simulink model "compiled_model"  (R2021a)
settings: Solver=VariableStepAuto  StartTime=0.0  StopTime=120  RelTol=1e-3
undefined symbols (not defined in the file or in its folder): sigbuilder_block
libraries: fuzblock x1, mpcadaslib x1
settings Model: Creator=uddin  LastModifiedBy=uddin

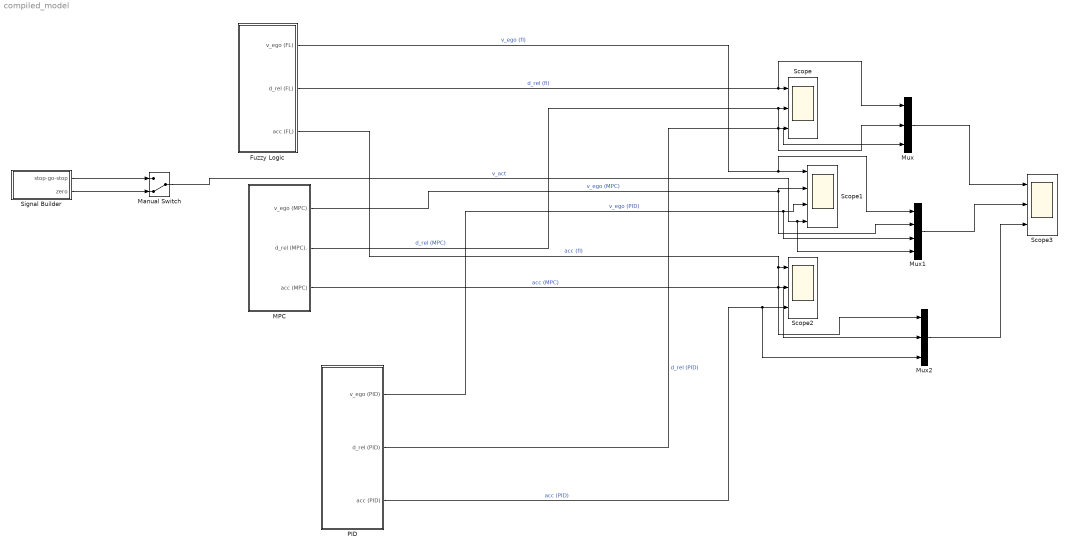
== system compiled_model ==
  Fuzzy Logic : Subsystem
  MPC : Subsystem
  Manual Switch : ManualSwitch  CurrentSetting=0
  Mux : Mux  Inputs=3
  Mux1 : Mux
  Mux2 : Mux  Inputs=3
  PID : Subsystem
  Scope : Scope  NumInputPorts=3
  Scope1 : Scope  NumInputPorts=4
  Scope2 : Scope  NumInputPorts=3
  Scope3 : Scope  NumInputPorts=3
  Signal Builder : Subsystem  Tag=STV Subsys  LoadFcn=sigbuilder_block('load');  StartFcn=sigbuilder_block('start');  StopFcn=sigbuilder_block('stop');  ClipboardFcn=sigbuilder_block('clipboard');  mask(Sigbuilder block){tuvar=[0:10]}
      mask help: Simulink:masks:SigbuilderBlock_MD
      mask init:
      | if ~strcmp(get_param(bdroot(gcbh),'SimulationStatus'),'stopped') tuvar = sigbuilder_block('maskInit'); end
      settings: CopyFcn=sigbuilder_block('copy');  DeleteFcn=sigbuilder_block('delete');  ModelCloseFcn=sigbuilder_block('modelClose');  PreSaveFcn=sigbuilder_block('preSave');  PauseFcn=sigbuilder_block('pause');  ContinueFcn=sigbuilder_block('continue');  NameChangeFcn=sigbuilder_block('namechange');  OpenFcn=sigbuilder_block('open',[393 134.4 550.8 400.2 ]);  CloseFcn=sigbuilder_block('close');
      mask Display: plot(0, 0, 100, 100,[2, 2, 32, 32, 2], [68, 8, 8, 68, 68],[32, 2], [38, 38], [32, 19, 2],[53, 60, 44], [32, 17, 17, 2],[16, 16, 31, 31]);txt = getActiveGroup(gcbh);text(2, 100, txt,'verticalAlignment', 'top');
  wires:
  Fuzzy Logic/2(d_rel (FL)) -> Mux/1, Scope/1  "d_rel (fl)"
  MPC/2(d_rel (MPC).) -> Mux/2, Scope/2  "d_rel (MPC)"
  PID/2(d_rel (PID)) -> Mux/3, Scope/3  "d_rel (PID)"
  Fuzzy Logic/1(v_ego (FL)) -> Mux1/1, Scope1/1  "v_ego (fl)"
  MPC/1(v_ego (MPC)) -> Mux1/2, Scope1/2  "v_ego (MPC)"
  PID/1(v_ego (PID)) -> Mux1/3, Scope1/3  "v_ego (PID)"
  Fuzzy Logic/3(acc (FL)) -> Mux2/1, Scope2/1  "acc (fl)"
  MPC/3(acc (MPC)) -> Mux2/2, Scope2/2  "acc (MPC)"
  PID/3(acc (PID)) -> Scope2/3, Mux2/3  "acc (PID)"
  Mux/1 -> Scope3/1
  Mux1/1 -> Scope3/2
  Mux2/1 -> Scope3/3
  Signal Builder/1(stop-go-stop) -> Manual Switch/1
  Signal Builder/2(zero) -> Manual Switch/2
  Manual Switch/1 -> Mux1/4, Scope1/4  "v_act"

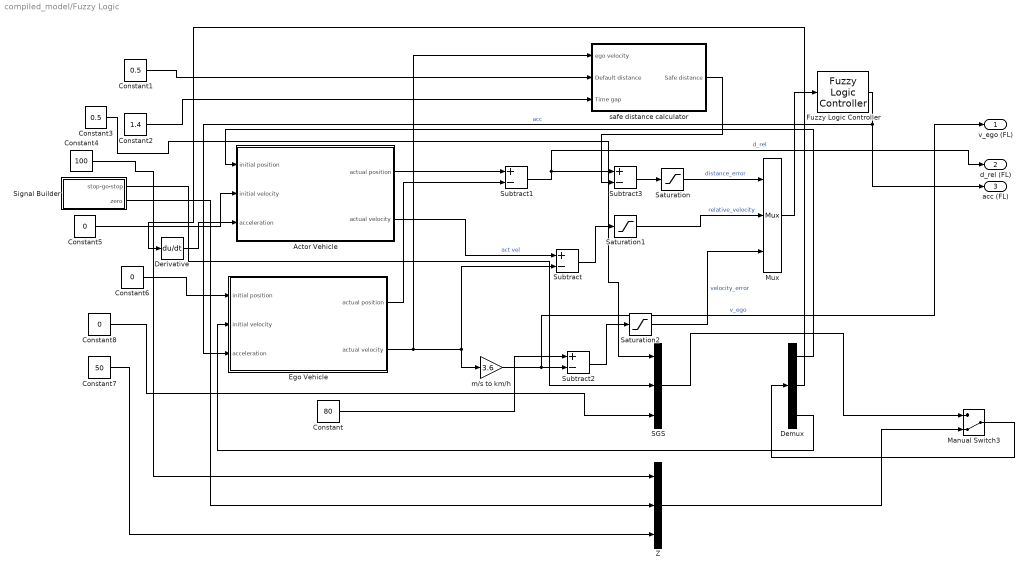
== system compiled_model/Fuzzy Logic ==
  Actor Vehicle : Subsystem
  Constant : Constant  Value=80  SampleTime=1
  Constant1 : Constant  Value=0.5  SampleTime=1
  Constant2 : Constant  Value=1.4  SampleTime=1
  Constant3 : Constant  Value=0.5  SampleTime=1
  Constant4 : Constant  Value=100  SampleTime=1
  Constant5 : Constant  Value=0  SampleTime=1
  Constant6 : Constant  Value=0  SampleTime=1
  Constant7 : Constant  Value=50  SampleTime=1
  Constant8 : Constant  Value=0  SampleTime=1
  Demux : Demux  Outputs=3
  Derivative : Derivative
  Ego Vehicle : Subsystem
  Fuzzy Logic Controller : fuzblock/Fuzzy Logic  Controller  FIS=self_created2  OutputSampleNumber=101  DataType=double  FuzzifiedInputs=off  RuleFiringStrengths=off  RuleOutputs=off  AggregatedOutputs=off  SimulateUsing=Interpreted execution  OutOfRangeInputValueMessage=none  NoRuleFiredMessage=none  EmptyOutputFuzzySetMessage=none
  Manual Switch3 : ManualSwitch  CurrentSetting=0
  Mux : Mux  Inputs=3
  SGS : Mux  Inputs=3
  Saturation : Saturate  UpperLimit=1  LowerLimit=-1  LinearizeAsGain=off  ZeroCross=off
  Saturation1 : Saturate  UpperLimit=1  LowerLimit=-1  LinearizeAsGain=off  ZeroCross=off
  Saturation2 : Saturate  UpperLimit=1  LowerLimit=-1  LinearizeAsGain=off  ZeroCross=off
  Signal Builder : Subsystem  Tag=STV Subsys  LoadFcn=sigbuilder_block('load');  StartFcn=sigbuilder_block('start');  StopFcn=sigbuilder_block('stop');  ClipboardFcn=sigbuilder_block('clipboard');  mask(Sigbuilder block){tuvar=[0:10]}
      mask help: Simulink:masks:SigbuilderBlock_MD
      mask init:
      | if ~strcmp(get_param(bdroot(gcbh),'SimulationStatus'),'stopped') tuvar = sigbuilder_block('maskInit'); end
      settings: CopyFcn=sigbuilder_block('copy');  DeleteFcn=sigbuilder_block('delete');  ModelCloseFcn=sigbuilder_block('modelClose');  PreSaveFcn=sigbuilder_block('preSave');  PauseFcn=sigbuilder_block('pause');  ContinueFcn=sigbuilder_block('continue');  NameChangeFcn=sigbuilder_block('namechange');  OpenFcn=sigbuilder_block('open',[393 134.4 550.8 400.2 ]);  CloseFcn=sigbuilder_block('close');
      mask Display: plot(0, 0, 100, 100,[2, 2, 32, 32, 2], [68, 8, 8, 68, 68],[32, 2], [38, 38], [32, 19, 2],[53, 60, 44], [32, 17, 17, 2],[16, 16, 31, 31]);txt = getActiveGroup(gcbh);text(2, 100, txt,'verticalAlignment', 'top');
  Subtract{,1..3} (4 alike) : Sum  Inputs=+-
  Z : Mux  Inputs=3
  m/s to km/h : Gain  Gain=3.6
  safe distance calculator : Subsystem
  v_ego (FL) : Outport
  d_rel (FL) : Outport  Port=2
  acc (FL) : Outport  Port=3
  wires:
  Actor Vehicle/2(actual velocity) -> Subtract/1  "act vel"
  Demux/2 -> Derivative/1
  m/s to km/h/1 -> v_ego (FL)/1, Subtract2/2  "v_ego"
  Subtract1/1 -> d_rel (FL)/1, Subtract3/1  "d_rel"
  Subtract3/1 -> Saturation/1
  Constant6/1 -> Ego Vehicle/1(initial position)
  Mux/1 -> Fuzzy Logic Controller/1
  Fuzzy Logic Controller/1 -> acc (FL)/1, Ego Vehicle/3(acceleration)  "acc"
  Ego Vehicle/1(actual position) -> Subtract1/2
  Constant3/1 -> SGS/1
  Saturation/1 -> Mux/1  "distance_error"
  Saturation1/1 -> Mux/2  "relative_velocity"
  Actor Vehicle/1(actual position) -> Subtract1/1
  Signal Builder/2(zero) -> Z/2
  safe distance calculator/1(Safe distance) -> Subtract3/2
  Ego Vehicle/2(actual velocity) -> safe distance calculator/1(ego velocity), m/s to km/h/1, Subtract/2
  Constant2/1 -> safe distance calculator/3(Time gap)
  Constant1/1 -> safe distance calculator/2(Default distance)
  Constant/1 -> Subtract2/1
  Constant7/1 -> Z/3
  Subtract2/1 -> Saturation2/1
  Constant4/1 -> Z/1
  Constant8/1 -> SGS/3
  Demux/1 -> Actor Vehicle/1(initial position)
  Derivative/1 -> Actor Vehicle/3(acceleration)
  Constant5/1 -> Actor Vehicle/2(initial velocity)
  Demux/3 -> Ego Vehicle/2(initial velocity)
  Saturation2/1 -> Mux/3  "velocity_error"
  Subtract/1 -> Saturation1/1
  Signal Builder/1(stop-go-stop) -> SGS/2
  SGS/1 -> Manual Switch3/1
  Manual Switch3/1 -> Demux/1
  Z/1 -> Manual Switch3/2

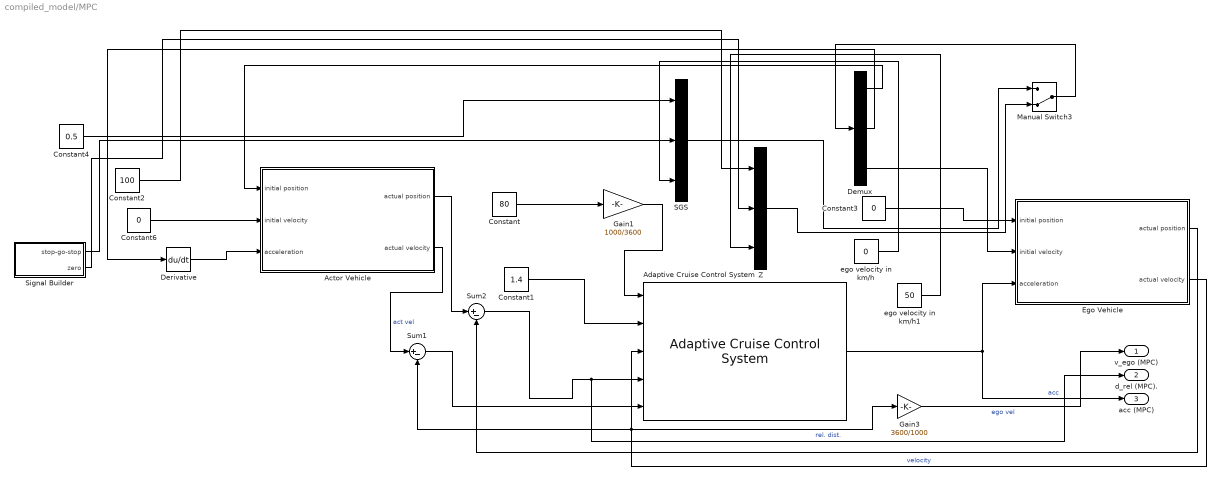
== system compiled_model/MPC ==
  Actor Vehicle : Subsystem
  Adaptive Cruise Control System : mpcadaslib/Adaptive Cruise Control System  EgoModel=tf(1,[0.5,1,0])  InitialEgoVelocity=50*1000/3600  DefaultSpacing=0.5  MaxVelocity=120*1000/3600  MinAcceleration=-3  amin_ext=off  MaxAcceleration=2  amax_ext=off  Ts=0.5  PredictionHorizon=25  ControllerBehavior=0.0  suboptimal=off  maxiter=20  datatypeopt=double  optmode=off  trackmode=off
  Constant : Constant  Value=80  SampleTime=1
  Constant1 : Constant  Value=1.4  SampleTime=1
  Constant2 : Constant  Value=100  SampleTime=1
  Constant3 : Constant  Value=0  SampleTime=1
  Constant4 : Constant  Value=0.5  SampleTime=1
  Constant6 : Constant  Value=0  SampleTime=1
  Demux : Demux  Outputs=3
  Derivative : Derivative
  Ego Vehicle : Subsystem
  Gain1 : Gain  Gain=1000/3600
  Gain3 : Gain  Gain=3600/1000
  Manual Switch3 : ManualSwitch  CurrentSetting=0
  SGS : Mux  Inputs=3
  Signal Builder : Subsystem  Tag=STV Subsys  LoadFcn=sigbuilder_block('load');  StartFcn=sigbuilder_block('start');  StopFcn=sigbuilder_block('stop');  ClipboardFcn=sigbuilder_block('clipboard');  mask(Sigbuilder block){tuvar=[0:10]}
      mask help: Simulink:masks:SigbuilderBlock_MD
      mask init:
      | if ~strcmp(get_param(bdroot(gcbh),'SimulationStatus'),'stopped') tuvar = sigbuilder_block('maskInit'); end
      settings: CopyFcn=sigbuilder_block('copy');  DeleteFcn=sigbuilder_block('delete');  ModelCloseFcn=sigbuilder_block('modelClose');  PreSaveFcn=sigbuilder_block('preSave');  PauseFcn=sigbuilder_block('pause');  ContinueFcn=sigbuilder_block('continue');  NameChangeFcn=sigbuilder_block('namechange');  OpenFcn=sigbuilder_block('open',[393 134.4 550.8 400.2 ]);  CloseFcn=sigbuilder_block('close');
      mask Display: plot(0, 0, 100, 100,[2, 2, 32, 32, 2], [68, 8, 8, 68, 68],[32, 2], [38, 38], [32, 19, 2],[53, 60, 44], [32, 17, 17, 2],[16, 16, 31, 31]);txt = getActiveGroup(gcbh);text(2, 100, txt,'verticalAlignment', 'top');
  Sum1 : Sum  Inputs=|+-
  Sum2 : Sum  Inputs=|+-
  Z : Mux  Inputs=3
  ego velocity in km/h : Constant  Value=0  SampleTime=1
  ego velocity in km/h1 : Constant  Value=50  SampleTime=1
  v_ego (MPC) : Outport
  d_rel (MPC). : Outport  Port=2
  acc (MPC) : Outport  Port=3
  wires:
  Sum1/1 -> Adaptive Cruise Control System/5
  Signal Builder/2(zero) -> Z/2
  Sum2/1 -> d_rel (MPC)./1, Adaptive Cruise Control System/4  "rel. dist."
  Actor Vehicle/2(actual velocity) -> Sum1/1  "act vel"
  Signal Builder/1(stop-go-stop) -> SGS/2
  Adaptive Cruise Control System/1 -> acc (MPC)/1, Ego Vehicle/3(acceleration)  "acc"
  Ego Vehicle/2(actual velocity) -> Gain3/1, Adaptive Cruise Control System/3, Sum1/2  "velocity"
  Gain3/1 -> v_ego (MPC)/1  "ego vel"
  Ego Vehicle/1(actual position) -> Sum2/2
  Constant3/1 -> Ego Vehicle/1(initial position)
  Gain1/1 -> Adaptive Cruise Control System/1
  Constant/1 -> Gain1/1
  Actor Vehicle/1(actual position) -> Sum2/1
  Constant1/1 -> Adaptive Cruise Control System/2
  Constant4/1 -> SGS/1
  Constant2/1 -> Z/1
  Demux/1 -> Actor Vehicle/1(initial position)
  Constant6/1 -> Actor Vehicle/2(initial velocity)
  Derivative/1 -> Actor Vehicle/3(acceleration)
  ego velocity in km/h/1 -> SGS/3
  ego velocity in km/h1/1 -> Z/3
  Demux/3 -> Ego Vehicle/2(initial velocity)
  SGS/1 -> Manual Switch3/1
  Manual Switch3/1 -> Demux/1
  Demux/2 -> Derivative/1
  Z/1 -> Manual Switch3/2

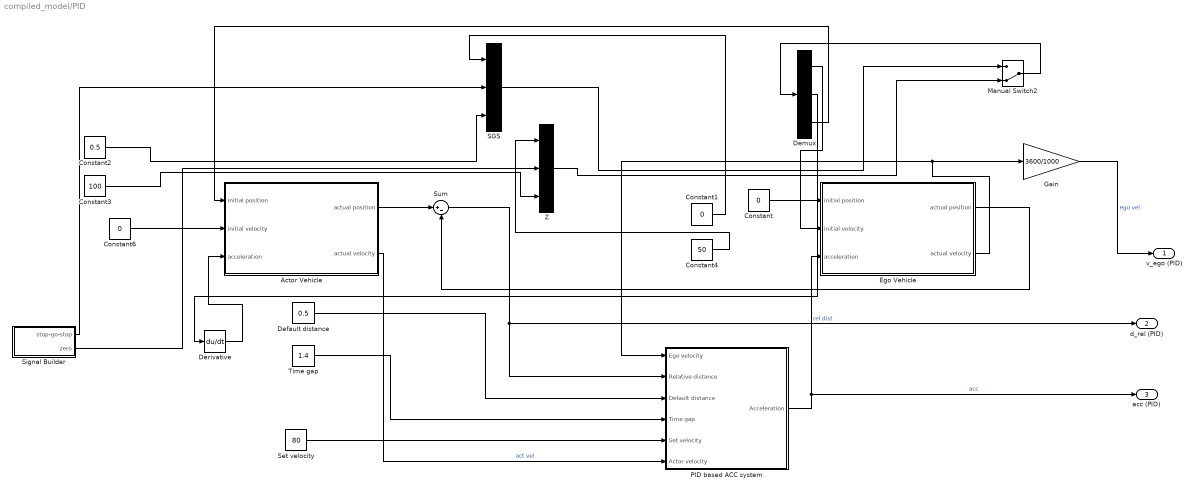
== system compiled_model/PID ==
  Actor Vehicle : Subsystem
  Constant : Constant  Value=0  SampleTime=.1
  Constant1 : Constant  Value=0  SampleTime=.1
  Constant2 : Constant  Value=0.5  SampleTime=.1
  Constant3 : Constant  Value=100  SampleTime=.1
  Constant4 : Constant  Value=50  SampleTime=.1
  Constant6 : Constant  Value=0  SampleTime=.1
  Default distance : Constant  Value=0.5  SampleTime=.1
  Demux : Demux  Outputs=3
  Derivative : Derivative
  Ego Vehicle : Subsystem
  Gain : Gain  Gain=3600/1000
  Manual Switch2 : ManualSwitch  CurrentSetting=0
  PID based ACC system : Subsystem
  SGS : Mux  Inputs=3
  Set velocity : Constant  Value=80  SampleTime=.1
  Signal Builder : Subsystem  Tag=STV Subsys  LoadFcn=sigbuilder_block('load');  StartFcn=sigbuilder_block('start');  StopFcn=sigbuilder_block('stop');  ClipboardFcn=sigbuilder_block('clipboard');  mask(Sigbuilder block){tuvar=[0:10]}
      mask help: Simulink:masks:SigbuilderBlock_MD
      mask init:
      | if ~strcmp(get_param(bdroot(gcbh),'SimulationStatus'),'stopped') tuvar = sigbuilder_block('maskInit'); end
      settings: CopyFcn=sigbuilder_block('copy');  DeleteFcn=sigbuilder_block('delete');  ModelCloseFcn=sigbuilder_block('modelClose');  PreSaveFcn=sigbuilder_block('preSave');  PauseFcn=sigbuilder_block('pause');  ContinueFcn=sigbuilder_block('continue');  NameChangeFcn=sigbuilder_block('namechange');  OpenFcn=sigbuilder_block('open',[393 134.4 550.8 400.2 ]);  CloseFcn=sigbuilder_block('close');
      mask Display: plot(0, 0, 100, 100,[2, 2, 32, 32, 2], [68, 8, 8, 68, 68],[32, 2], [38, 38], [32, 19, 2],[53, 60, 44], [32, 17, 17, 2],[16, 16, 31, 31]);txt = getActiveGroup(gcbh);text(2, 100, txt,'verticalAlignment', 'top');
  Sum : Sum  Inputs=|+-
  Time gap : Constant  Value=1.4  SampleTime=.1
  Z : Mux  Inputs=3
  v_ego (PID) : Outport
  d_rel (PID) : Outport  Port=2
  acc (PID) : Outport  Port=3
  wires:
  Signal Builder/2(zero) -> Z/2
  Actor Vehicle/2(actual velocity) -> PID based ACC system/6(Actor velocity)  "act vel"
  Constant/1 -> Ego Vehicle/1(initial position)
  PID based ACC system/1(Acceleration) -> acc (PID)/1, Ego Vehicle/3(acceleration)  "acc"
  Default distance/1 -> PID based ACC system/3(Default distance)
  Sum/1 -> PID based ACC system/2(Relative distance), d_rel (PID)/1  "rel dist"
  Actor Vehicle/1(actual position) -> Sum/1
  Signal Builder/1(stop-go-stop) -> SGS/2
  Time gap/1 -> PID based ACC system/4(Time gap)
  Set velocity/1 -> PID based ACC system/5(Set velocity)
  Ego Vehicle/2(actual velocity) -> PID based ACC system/1(Ego velocity), Gain/1
  Ego Vehicle/1(actual position) -> Sum/2
  Gain/1 -> v_ego (PID)/1  "ego vel"
  Constant6/1 -> Actor Vehicle/2(initial velocity)
  Demux/2 -> Derivative/1
  Derivative/1 -> Actor Vehicle/3(acceleration)
  Constant2/1 -> SGS/3
  Demux/3 -> Actor Vehicle/1(initial position)
  SGS/1 -> Manual Switch2/1
  Z/1 -> Manual Switch2/2
  Manual Switch2/1 -> Demux/1
  Constant3/1 -> Z/3
  Constant4/1 -> Z/1
  Constant1/1 -> SGS/1
  Demux/1 -> Ego Vehicle/2(initial velocity)

== system compiled_model/Signal Builder ==
  Demux : Demux  Tag=STV Demux  Outputs=2
      settings: DisplayOption=none
  FromWs : FromWorkspace  Tag=STV FromWs  VariableName=tuvar
      SigBuilderData=|
      | common.afterFinalStr = 'Extrapolate'
      | common.sampleTime = 0
      | dataSet.timeRange = [0 30]
      | dataSet.name = 'Group 1'
      | sbobj.Groups.Name = 'Group 1'
      | sbobj.Groups.Signals(1).Name = 'stop-go-stop'
      | sbobj.Groups.Signals(1).XData = [0 5 10 20 25 30]
      | sbobj.Groups.Signals(1).YData = [0 0 2 2 0 0]
      | sbobj.Groups.Signals(2).Name = 'zero'
      | sbobj.Groups.Signals(2).XData = [0 30]
      | sbobj.Groups.Signals(2).YData = [0 0]
      | sbobj.Groups.TimeRange = [0 30]
  stop-go-stop : Outport  Tag=STV Outport
  zero : Outport  Tag=STV Outport  Port=2
  wires:
  FromWs/1 -> Demux/1
  Demux/1 -> stop-go-stop/1
  Demux/2 -> zero/1

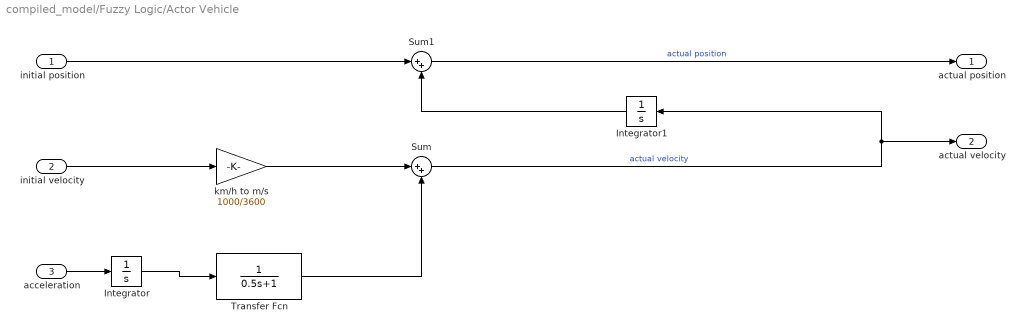
== system compiled_model/Fuzzy Logic/Actor Vehicle ==
  initial position : Inport
  initial velocity : Inport  Port=2
  acceleration : Inport  Port=3
  Integrator : Integrator  ZeroCross=off
  Integrator1 : Integrator  ZeroCross=off
  Sum : Sum  Inputs=|++
  Sum1 : Sum  Inputs=|++
  Transfer Fcn : TransferFcn  Denominator=[0.5 1]
  km/h to m/s : Gain  Gain=1000/3600
  actual position : Outport
  actual velocity : Outport  Port=2
  wires:
  km/h to m/s/1 -> Sum/1
  initial velocity/1 -> km/h to m/s/1
  Transfer Fcn/1 -> Sum/2
  Integrator/1 -> Transfer Fcn/1
  Integrator1/1 -> Sum1/2
  initial position/1 -> Sum1/1
  acceleration/1 -> Integrator/1
  Sum/1 -> Integrator1/1, actual velocity/1  "actual velocity"
  Sum1/1 -> actual position/1  "actual position"

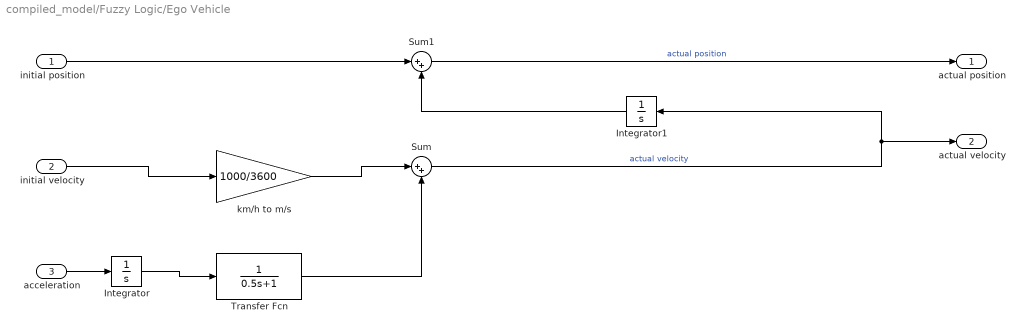
== system compiled_model/Fuzzy Logic/Ego Vehicle ==
  initial position : Inport
  initial velocity : Inport  Port=2
  acceleration : Inport  Port=3
  Integrator : Integrator  ZeroCross=off
  Integrator1 : Integrator  ZeroCross=off
  Sum : Sum  Inputs=|++
  Sum1 : Sum  Inputs=|++
  Transfer Fcn : TransferFcn  Denominator=[0.5 1]
  km/h to m/s : Gain  Gain=1000/3600
  actual position : Outport
  actual velocity : Outport  Port=2
  wires:
  Sum1/1 -> actual position/1  "actual position"
  Sum/1 -> actual velocity/1, Integrator1/1  "actual velocity"
  acceleration/1 -> Integrator/1
  initial position/1 -> Sum1/1
  Integrator1/1 -> Sum1/2
  Integrator/1 -> Transfer Fcn/1
  Transfer Fcn/1 -> Sum/2
  initial velocity/1 -> km/h to m/s/1
  km/h to m/s/1 -> Sum/1

== system compiled_model/Fuzzy Logic/Signal Builder ==
  Demux : Demux  Tag=STV Demux  Outputs=2
      settings: DisplayOption=none
  FromWs : FromWorkspace  Tag=STV FromWs  VariableName=tuvar
      SigBuilderData=|
      | common.afterFinalStr = 'Extrapolate'
      | common.sampleTime = 0
      | dataSet.timeRange = [0 30]
      | dataSet.name = 'Group 1'
      | sbobj.Groups.Name = 'Group 1'
      | sbobj.Groups.Signals(1).Name = 'stop-go-stop'
      | sbobj.Groups.Signals(1).XData = [0 5 10 20 25 30]
      | sbobj.Groups.Signals(1).YData = [0 0 2 2 0 0]
      | sbobj.Groups.Signals(2).Name = 'zero'
      | sbobj.Groups.Signals(2).XData = [0 30]
      | sbobj.Groups.Signals(2).YData = [0 0]
      | sbobj.Groups.TimeRange = [0 30]
  stop-go-stop : Outport  Tag=STV Outport
  zero : Outport  Tag=STV Outport  Port=2
  wires:
  FromWs/1 -> Demux/1
  Demux/1 -> stop-go-stop/1
  Demux/2 -> zero/1

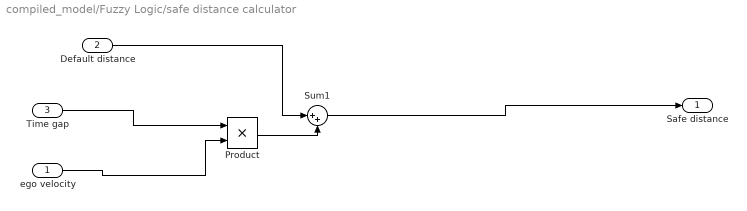
== system compiled_model/Fuzzy Logic/safe distance calculator ==
  ego velocity : Inport
  Default distance : Inport  Port=2
  Time gap : Inport  Port=3
  Product : Product
  Sum1 : Sum  Inputs=|++
  Safe distance : Outport
  wires:
  Product/1 -> Sum1/2
  Sum1/1 -> Safe distance/1
  Time gap/1 -> Product/1
  Default distance/1 -> Sum1/1
  ego velocity/1 -> Product/2

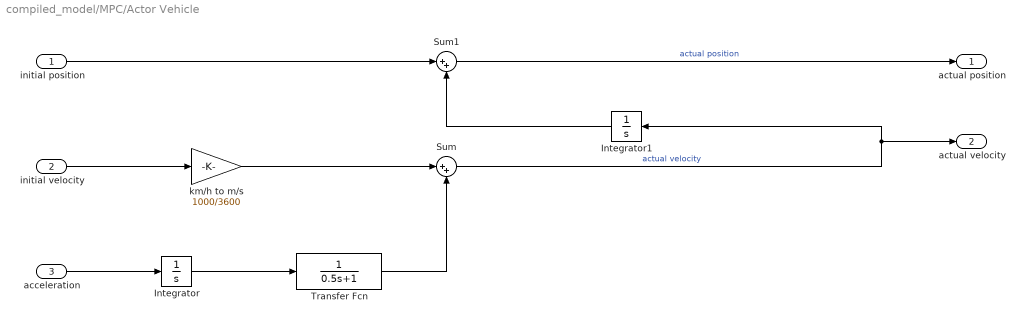
== system compiled_model/MPC/Actor Vehicle ==
  initial position : Inport
  initial velocity : Inport  Port=2
  acceleration : Inport  Port=3
  Integrator : Integrator  ZeroCross=off
  Integrator1 : Integrator  ZeroCross=off
  Sum : Sum  Inputs=|++
  Sum1 : Sum  Inputs=|++
  Transfer Fcn : TransferFcn  Denominator=[0.5 1]
  km/h to m/s : Gain  Gain=1000/3600
  actual position : Outport
  actual velocity : Outport  Port=2
  wires:
  Integrator1/1 -> Sum1/2
  initial position/1 -> Sum1/1
  acceleration/1 -> Integrator/1
  Sum/1 -> Integrator1/1, actual velocity/1  "actual velocity"
  Sum1/1 -> actual position/1  "actual position"
  Integrator/1 -> Transfer Fcn/1
  Transfer Fcn/1 -> Sum/2
  initial velocity/1 -> km/h to m/s/1
  km/h to m/s/1 -> Sum/1

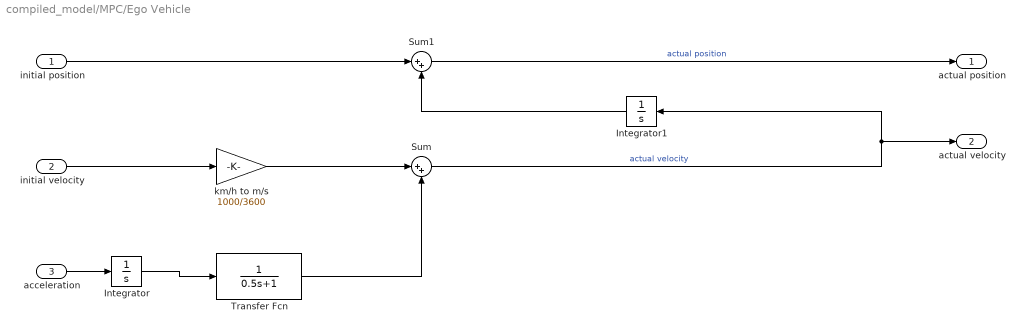
== system compiled_model/MPC/Ego Vehicle ==
  initial position : Inport
  initial velocity : Inport  Port=2
  acceleration : Inport  Port=3
  Integrator : Integrator  ZeroCross=off
  Integrator1 : Integrator  ZeroCross=off
  Sum : Sum  Inputs=|++
  Sum1 : Sum  Inputs=|++
  Transfer Fcn : TransferFcn  Denominator=[0.5 1]
  km/h to m/s : Gain  Gain=1000/3600
  actual position : Outport
  actual velocity : Outport  Port=2
  wires:
  Sum1/1 -> actual position/1  "actual position"
  Sum/1 -> actual velocity/1, Integrator1/1  "actual velocity"
  acceleration/1 -> Integrator/1
  initial position/1 -> Sum1/1
  Integrator1/1 -> Sum1/2
  Integrator/1 -> Transfer Fcn/1
  Transfer Fcn/1 -> Sum/2
  initial velocity/1 -> km/h to m/s/1
  km/h to m/s/1 -> Sum/1

== system compiled_model/MPC/Signal Builder ==
  Demux : Demux  Tag=STV Demux  Outputs=2
      settings: DisplayOption=none
  FromWs : FromWorkspace  Tag=STV FromWs  VariableName=tuvar
      SigBuilderData=|
      | common.afterFinalStr = 'Extrapolate'
      | common.sampleTime = 0
      | dataSet.timeRange = [0 30]
      | dataSet.name = 'Group 1'
      | sbobj.Groups.Name = 'Group 1'
      | sbobj.Groups.Signals(1).Name = 'stop-go-stop'
      | sbobj.Groups.Signals(1).XData = [0 5 10 20 25 30]
      | sbobj.Groups.Signals(1).YData = [0 0 2 2 0 0]
      | sbobj.Groups.Signals(2).Name = 'zero'
      | sbobj.Groups.Signals(2).XData = [0 30]
      | sbobj.Groups.Signals(2).YData = [0 0]
      | sbobj.Groups.TimeRange = [0 30]
  stop-go-stop : Outport  Tag=STV Outport
  zero : Outport  Tag=STV Outport  Port=2
  wires:
  FromWs/1 -> Demux/1
  Demux/1 -> stop-go-stop/1
  Demux/2 -> zero/1

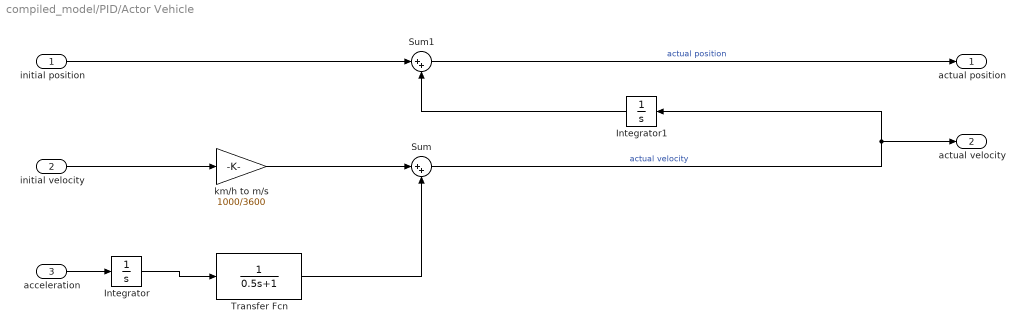
== system compiled_model/PID/Actor Vehicle ==
  initial position : Inport
  initial velocity : Inport  Port=2
  acceleration : Inport  Port=3
  Integrator : Integrator
  Integrator1 : Integrator
  Sum : Sum  Inputs=|++
  Sum1 : Sum  Inputs=|++
  Transfer Fcn : TransferFcn  Denominator=[0.5 1]
  km/h to m/s : Gain  Gain=1000/3600
  actual position : Outport
  actual velocity : Outport  Port=2
  wires:
  km/h to m/s/1 -> Sum/1
  initial velocity/1 -> km/h to m/s/1
  Transfer Fcn/1 -> Sum/2
  Integrator/1 -> Transfer Fcn/1
  Integrator1/1 -> Sum1/2
  initial position/1 -> Sum1/1
  acceleration/1 -> Integrator/1
  Sum/1 -> Integrator1/1, actual velocity/1  "actual velocity"
  Sum1/1 -> actual position/1  "actual position"

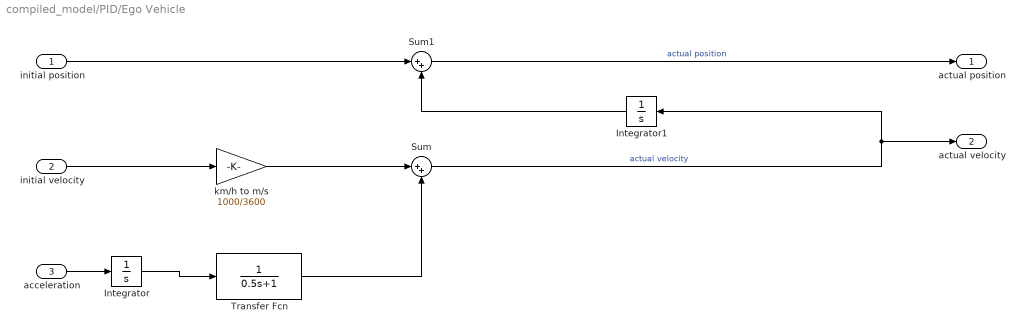
== system compiled_model/PID/Ego Vehicle ==
  initial position : Inport
  initial velocity : Inport  Port=2
  acceleration : Inport  Port=3
  Integrator : Integrator
  Integrator1 : Integrator
  Sum : Sum  Inputs=|++
  Sum1 : Sum  Inputs=|++
  Transfer Fcn : TransferFcn  Denominator=[0.5 1]
  km/h to m/s : Gain  Gain=1000/3600
  actual position : Outport
  actual velocity : Outport  Port=2
  wires:
  Sum1/1 -> actual position/1  "actual position"
  Sum/1 -> actual velocity/1, Integrator1/1  "actual velocity"
  acceleration/1 -> Integrator/1
  initial position/1 -> Sum1/1
  Integrator1/1 -> Sum1/2
  Integrator/1 -> Transfer Fcn/1
  Transfer Fcn/1 -> Sum/2
  initial velocity/1 -> km/h to m/s/1
  km/h to m/s/1 -> Sum/1

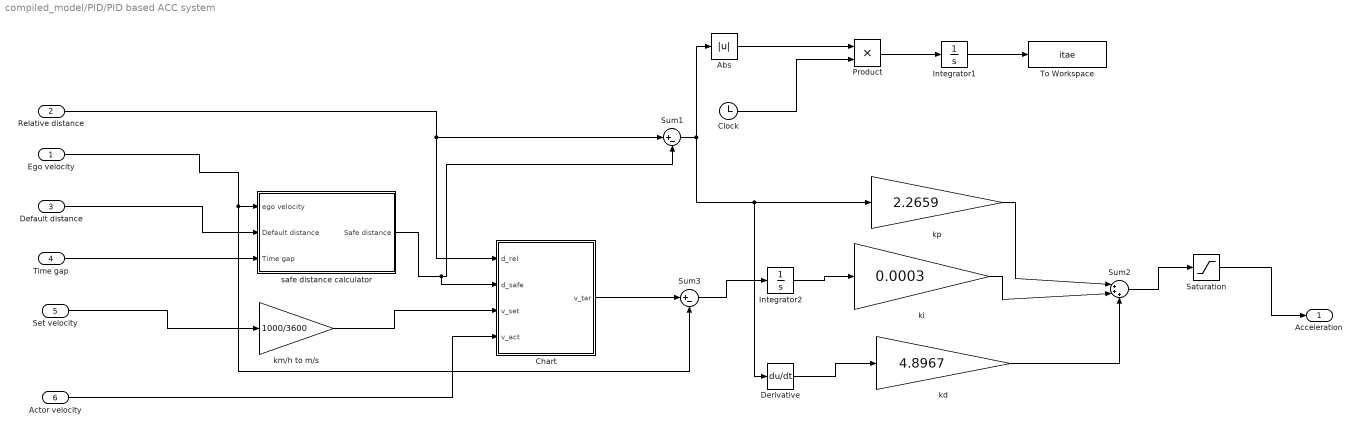
== system compiled_model/PID/PID based ACC system ==
  Ego velocity : Inport
  Relative distance : Inport  Port=2
  Default distance : Inport  Port=3
  Time gap : Inport  Port=4
  Set velocity : Inport  Port=5
  Actor velocity : Inport  Port=6
  Abs : Abs  ZeroCross=off
  Chart : Stateflow chart  TreatAsAtomicUnit=on
  Clock : Clock
  Derivative : Derivative
  Integrator1 : Integrator
  Integrator2 : Integrator
  Product : Product
  Saturation : Saturate  UpperLimit=2  LowerLimit=-3  LinearizeAsGain=off  ZeroCross=off
  Sum1 : Sum  Inputs=|+-
  Sum2 : Sum  Inputs=|+++
  Sum3 : Sum  Inputs=|+-
  To Workspace : ToWorkspace  VariableName=itae  SampleTime=1
      settings: Save2DSignal=2-D array (concatenate along first dimension)
  kd : Gain  Gain=4.8967
  ki : Gain  Gain=0.0003
  km/h to m/s : Gain  Gain=1000/3600
  kp : Gain  Gain=2.2659
  safe distance calculator : Subsystem
  Acceleration : Outport
  wires:
  Default distance/1 -> safe distance calculator/2(Default distance)
  Set velocity/1 -> km/h to m/s/1
  Time gap/1 -> safe distance calculator/3(Time gap)
  Ego velocity/1 -> safe distance calculator/1(ego velocity), Sum3/2
  ki/1 -> Sum2/2
  kp/1 -> Sum2/1
  Relative distance/1 -> Chart/1(d_rel), Sum1/1
  safe distance calculator/1(Safe distance) -> Sum1/2, Chart/2(d_safe)
  km/h to m/s/1 -> Chart/3(v_set)
  Actor velocity/1 -> Chart/4(v_act)
  Sum1/1 -> Derivative/1, kp/1, Abs/1
  Abs/1 -> Product/1
  Derivative/1 -> kd/1
  kd/1 -> Sum2/3
  Chart/1(v_tar) -> Sum3/1
  Integrator2/1 -> ki/1
  Sum2/1 -> Saturation/1
  Saturation/1 -> Acceleration/1
  Product/1 -> Integrator1/1
  Integrator1/1 -> To Workspace/1
  Clock/1 -> Product/2
  Sum3/1 -> Integrator2/1

== system compiled_model/PID/Signal Builder ==
  Demux : Demux  Tag=STV Demux  Outputs=2
      settings: DisplayOption=none
  FromWs : FromWorkspace  Tag=STV FromWs  VariableName=tuvar
      SigBuilderData=|
      | common.afterFinalStr = 'Extrapolate'
      | common.sampleTime = 0
      | dataSet.timeRange = [0 30]
      | dataSet.name = 'Group 1'
      | sbobj.Groups.Name = 'Group 1'
      | sbobj.Groups.Signals(1).Name = 'stop-go-stop'
      | sbobj.Groups.Signals(1).XData = [0 5 10 20 25 30]
      | sbobj.Groups.Signals(1).YData = [0 0 2 2 0 0]
      | sbobj.Groups.Signals(2).Name = 'zero'
      | sbobj.Groups.Signals(2).XData = [0 30]
      | sbobj.Groups.Signals(2).YData = [0 0]
      | sbobj.Groups.TimeRange = [0 30]
  stop-go-stop : Outport  Tag=STV Outport
  zero : Outport  Tag=STV Outport  Port=2
  wires:
  FromWs/1 -> Demux/1
  Demux/1 -> stop-go-stop/1
  Demux/2 -> zero/1

== system compiled_model/PID/PID based ACC system/safe distance calculator ==
  ego velocity : Inport
  Default distance : Inport  Port=2
  Time gap : Inport  Port=3
  Product : Product
  Sum1 : Sum  Inputs=|++
  Safe distance : Outport
  wires:
  Product/1 -> Sum1/2
  Sum1/1 -> Safe distance/1
  Time gap/1 -> Product/1
  Default distance/1 -> Sum1/1
  ego velocity/1 -> Product/2

== stateflow chart compiled_model/PID/PID based ACC system/Chart ==
  (default) -> (junction 7)
  (junction 7) -> (junction 8) [order 1] : [d_rel>d_safe]
  (junction 7) -> (junction 9) [order 2] : {v_tar=v_act;}
  (junction 8) -> (junction 10) : {v_tar=v_set;}
  (junction 10) -> (junction 9)
  (junction 9) -> (junction 11)
  data: d_rel input; d_safe input; v_set input; v_act input; v_tar output
